simulink model "stateflow_transitions"  (R2015b)
settings: Solver=VariableStepAuto  StartTime=0.0  StopTime=10.0  RelTol=1e-3
settings Model: Creator=ladmin  LastModifiedBy=ladmin

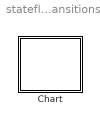
== system stateflow_transitions ==
  Chart : Stateflow chart  TreatAsAtomicUnit=on

== stateflow chart stateflow_transitions/Chart ==
  state ABC
    state DEF
  state GHI
  ABC -> GHI : [Bigger Label 2]
  (default) -> ABC [order 2]
  (default) -> (junction 4) [order 1] : [big arrow head]
  GHI -> ABC : MyLabel
